simulink model "Xbox_collision_final"  (R2018b)
settings: Solver=FixedStepAuto  StartTime=0.0  StopTime=inf  FixedStep=Ts  RelTol=1e-3  EnableMultiTasking=on
PreLoadFcn:
  | config
InitFcn:
  | gb_params_obs
values from neighbouring files (symbols this model uses):
  A1 = [0, 0, 1, 0 ... (first row only)    [gb_load.m]    (also in gb_params_obs.m; model.m)
  A2 = [0   1 ... (first row only)    [gb_load.m]    (also in gb_params_obs.m; model.m)
  ag = 0.8    [gb_load.m]    (also in gb_params_obs.m; model.m)
  B1 = [0;0;2*alpha*(g2+g4)/g5; -2*alpha*(g2+g3)/g5]    [gb_load.m]    (also in gb_params_obs.m; model.m)
  B2 = [0 ... (first row only)    [gb_load.m]    (also in gb_params_obs.m; model.m)
  C1 = eye(4)    [gb_load.m]    (also in gb_params_obs.m; model.m = [1, -1, 0, 0)
  C1o = [1, -1, 0, 0 ... (first row only)    [gb_load.m]    (also in gb_params_obs.m)
  C2 = eye(2)    [gb_load.m]    (also in gb_params_obs.m; model.m = [1,0])
  C2o = [1,0]    [gb_load.m]    (also in gb_params_obs.m)
  Cg = [0,0,0,1,0,0]    [gb_load.m]    (also in gb_params_obs.m; model.m)
  Cm = [1,-1,0,0,1,0 ... (first row only)    [gb_load.m]    (also in gb_params_obs.m; model.m = [1,-1,0,0,W/(2*R),0)
  D1 = zeros(4, 1)    [gb_load.m]    (also in gb_params_obs.m)
  D2 = zeros(2,1)    [gb_load.m]    (also in gb_params_obs.m)
  EV3 = 0    [setup.m]
  K1i = lqrd(A1i, B1i, Q1i, R1i, Ts)    [gb_load.m]    (also in gb_params_obs.m)
  K2 = A2(2,2)^2/(4*B2(2,1))    [gb_load.m]    (also in gb_params_obs.m)
  kest = ss(ssd.A - L2t*ssd.C, [ssd.B L2t], ssd.C, zeros(2,3))    [gb_params_obs.m]
  R = 0.027    [gb_load.m]    (also in gb_params_obs.m; model.m; paramsCW2_v8.m = 0.01)
  Ts = 0.002    [gb_load.m]    (also in gb_params_obs.m; model.m; paramsCW2_v8.m = 0.004)
undefined symbols (not defined in the file or in its folder): DiscIntNeverNeededParam
libraries: legoev3lib x7, simulink_extras x6, simulink x1, shared_linuxserviceslib x1
settings Model: SimulationMode=external  ExtModeTrigDuration=2  Creator=thh206  LastModifiedBy=gazea
settings SolverCC: PositivePriorityOrder=on
settings OptimizationCC: EnhancedBackFolding=on  PassReuseOutputArgsAs=Individual arguments  MaxStackSize=64  OptimizeBlockOrder=speed  DifferentSizesBufferReuse=on  OptimizationCustomize=off
settings DebuggingCC: ParameterTunabilityLossMsg=error  LibraryContextMissingDiagnostic=none
settings HardwareCC: ProdBitPerPointer=32  ProdBitPerSizeT=32  ProdBitPerPtrDiffT=32  ProdLargestAtomicInteger=Long  ProdWordSize=32  ProdHWDeviceType=ARM Compatible->ARM 9
settings SFSimCC: SimUseLocalCustomCode=off  MATLABDynamicMemAlloc=off
settings RTWCC: SystemTargetFile=ert.tlc  HardwareBoard=LEGO MINDSTORMS EV3  TLCOptions="-aInlineSetEventsForThisBaseRateFcn=TLC_FALSE -aSuppressMultiTaskScheduler=TLC_FALSE  -aRateBasedStepFcn=0"  TemplateMakefile=ert_default_tmf  GenerateReport=on  RTWUseLocalCustomCode=off  Toolchain=Sourcery G++ Lite v2009q3  IncludeHyperlinkInReport=on  LaunchReport=on  GenerateTraceInfo=on  GenerateTraceReport=on  GenerateTraceReportSl=on  GenerateTraceReportSf=on  GenerateTraceReportEml=on
settings CodeAppCC: ForceParamTrailComments=on  IgnoreCustomStorageClasses=off  OperatorAnnotations=on  SimulinkDataObjDesc=on  SFDataObjDesc=on  InsertBlockDesc=on
settings ERTTargetCC: SupportContinuousTime=on  SupportVariableSizeSignals=on

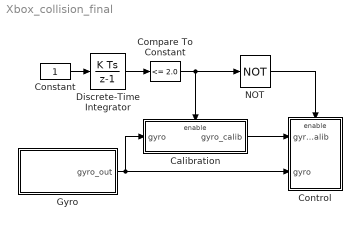
== system Xbox_collision_final ==
  Calibration : Subsystem
  Compare To Constant : simulink/Logic and Bit Operations/Compare To Constant  relop=<=  const=2.0  OutDataTypeStr=boolean
  Constant : Constant
  Control : Subsystem
  Discrete-Time Integrator : DiscreteIntegrator  SampleTime=Ts  ICPrevOutput=DiscIntNeverNeededParam  ICPrevScaledInput=DiscIntNeverNeededParam
  Gyro : Subsystem  Variant=on  VariantControl=Variant1
  NOT : Logic  Operator=NOT  IconShape=distinctive  AllPortsSameDT=off  OutDataTypeStr=boolean
  wires:
  Gyro/1(" gyro_out") -> Calibration/1(gyro), Control/2(gyro)
  Discrete-Time Integrator/1 -> Compare To Constant/1
  Compare To Constant/1 -> Calibration/Enable, NOT/1
  Constant/1 -> Discrete-Time Integrator/1
  NOT/1 -> Control/Enable
  Calibration/1(gyro_calib) -> Control/1(gyro_calib)

== system Xbox_collision_final/Calibration ==
  gyro : Inport
  Enable : EnablePort
  Gain1 : Gain  Gain=1-ag  OutDataTypeStr=Inherit: Same as input  ParamDataTypeStr=Inherit: Same as input
  Gain4 : Gain  Gain=ag  OutDataTypeStr=Inherit: Same as input  ParamDataTypeStr=Inherit: Same as input
  Scope : Scope
  Sum : Sum  Inputs=|++  OutDataTypeStr=Inherit: Same as first input
  Unit Delay : UnitDelay  InitialCondition=[0]  SampleTime=Ts
  gyro_calib : Outport
  wires:
  Unit Delay/1 -> Gain4/1
  Gain4/1 -> Sum/1
  Gain1/1 -> Sum/2
  Sum/1 -> Scope/1, gyro_calib/1, Unit Delay/1
  gyro/1 -> Gain1/1

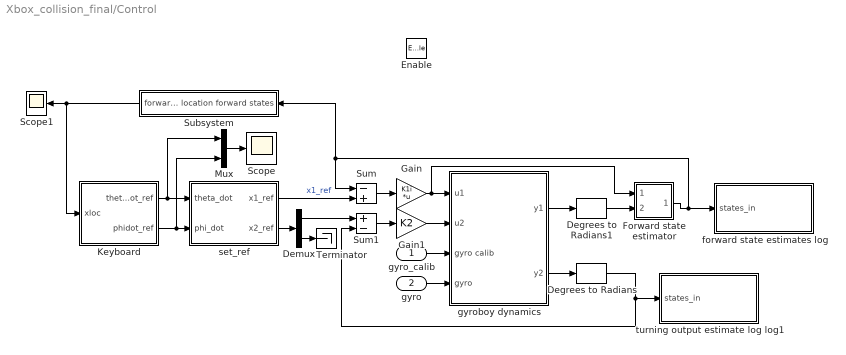
== system Xbox_collision_final/Control ==
  gyro_calib : Inport
  gyro : Inport  Port=2
  Enable : EnablePort
  Degrees to Radians : simulink_extras/Transformations/Degrees to Radians
  Degrees to Radians1 : simulink_extras/Transformations/Degrees to Radians
  Demux : Demux  Outputs=2
  Forward state estimator : Subsystem
  Gain : Gain  Gain=K1i  Multiplication=Matrix(K*u)
  Gain1 : Gain  Gain=K2
  Keyboard : Subsystem
  Mux : Mux  Inputs=2
  Scope : Scope
  Scope1 : Scope
  Subsystem : Subsystem
  Sum : Sum  Inputs=-+
  Sum1 : Sum  Inputs=+-
  Terminator : Terminator
  forward state estimates log : Subsystem  Variant=on  VariantControl=Variant1
  gyroboy dynamics : Subsystem  Variant=on  VariantControl=Variant1
  set_ref : Subsystem
  turning output estimate log log1 : Subsystem  Variant=on  VariantControl=Variant1
  wires:
  Keyboard/2(phidot_ref) -> Mux/2, set_ref/2(phi_dot)
  Keyboard/1(thetadot_ref) -> Mux/1, set_ref/1(theta_dot)
  Degrees to Radians/1 -> turning output estimate log log1/1(states_in), Sum1/2
  Gain/1 -> Forward state estimator/1(u1), gyroboy dynamics/1(u1)
  Gain1/1 -> gyroboy dynamics/2(u2)
  Sum1/1 -> Gain1/1
  gyroboy dynamics/2(y2) -> Degrees to Radians/1
  Mux/1 -> Scope/1
  set_ref/2(x2_ref) -> Demux/1
  Degrees to Radians1/1 -> Forward state estimator/2(y1)
  gyroboy dynamics/1(y1) -> Degrees to Radians1/1
  Demux/1 -> Sum1/1
  Sum/1 -> Gain/1
  Forward state estimator/1(x1e) -> forward state estimates log/1(states_in), Subsystem/1(forward states), Sum/1
  Demux/2 -> Terminator/1
  set_ref/1(x1_ref) -> Sum/2  "x1_ref"
  gyro_calib/1 -> gyroboy dynamics/3(gyro calib)
  Subsystem/1(forward location) -> Keyboard/1(xloc), Scope1/1
  gyro/1 -> gyroboy dynamics/4(gyro)

== system Xbox_collision_final/Gyro ==
  EV3 : Subsystem  VariantControl=HW == 1
  State-space : Subsystem  VariantControl=(default)
  " gyro_out" : Outport

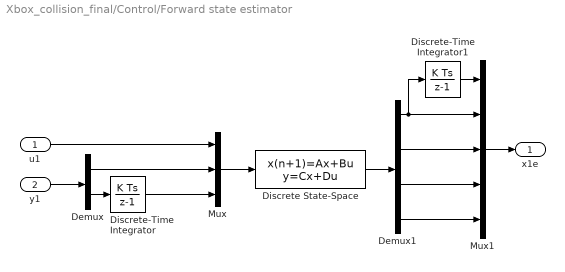
== system Xbox_collision_final/Control/Forward state estimator ==
  u1 : Inport
  y1 : Inport  Port=2
  Demux : Demux  Outputs=2
  Demux1 : Demux
  Discrete State-Space : DiscreteStateSpace  A=kest.A  B=kest.B  C=eye(4)  D=zeros(4,3)  InitialCondition=[0;0;0;0]  SampleTime=Ts
  Discrete-Time Integrator : DiscreteIntegrator  SampleTime=Ts  ICPrevOutput=DiscIntNeverNeededParam  ICPrevScaledInput=DiscIntNeverNeededParam
  Discrete-Time Integrator1 : DiscreteIntegrator  SampleTime=Ts  ICPrevOutput=DiscIntNeverNeededParam  ICPrevScaledInput=DiscIntNeverNeededParam
  Mux : Mux  Inputs=3
  Mux1 : Mux  Inputs=5
  x1e : Outport
  wires:
  y1/1 -> Demux/1
  Demux/2 -> Discrete-Time Integrator/1
  Discrete-Time Integrator/1 -> Mux/3
  Demux/1 -> Mux/2
  u1/1 -> Mux/1
  Mux/1 -> Discrete State-Space/1
  Demux1/4 -> Mux1/5
  Discrete-Time Integrator1/1 -> Mux1/1
  Demux1/1 -> Mux1/2, Discrete-Time Integrator1/1
  Demux1/2 -> Mux1/3
  Demux1/3 -> Mux1/4
  Mux1/1 -> x1e/1
  Discrete State-Space/1 -> Demux1/1

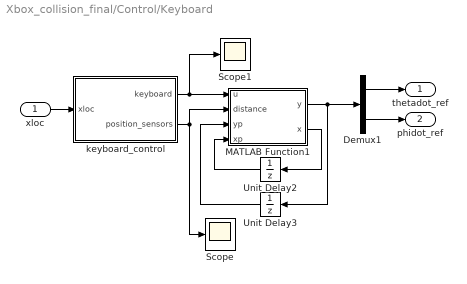
== system Xbox_collision_final/Control/Keyboard ==
  xloc : Inport
  Demux1 : Demux  Outputs=2
  MATLAB Function1 : MATLAB Function  TreatAsAtomicUnit=on
  Scope : Scope
  Scope1 : Scope
  Unit Delay2 : UnitDelay  InitialCondition=[0;0]  SampleTime=-1
  Unit Delay3 : UnitDelay  InitialCondition=[0;0]  SampleTime=-1
  keyboard_control : Subsystem  Variant=on  VariantControl=Variant1
  thetadot_ref : Outport
  phidot_ref : Outport  Port=2
  wires:
  Demux1/1 -> thetadot_ref/1
  MATLAB Function1/1(y) -> Demux1/1, Unit Delay3/1
  Unit Delay3/1 -> MATLAB Function1/3(yp)
  MATLAB Function1/2(x) -> Unit Delay2/1
  Unit Delay2/1 -> MATLAB Function1/4(xp)
  Demux1/2 -> phidot_ref/1
  keyboard_control/2(position_sensors) -> MATLAB Function1/2(distance), Scope/1
  keyboard_control/1(keyboard) -> MATLAB Function1/1(u), Scope1/1
  xloc/1 -> keyboard_control/1(xloc)

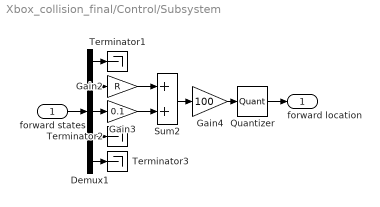
== system Xbox_collision_final/Control/Subsystem ==
  forward states : Inport
  Demux1 : Demux  Outputs=5
  Gain2 : Gain  Gain=R
  Gain3 : Gain  Gain=0.1
  Gain4 : Gain  Gain=100
  Quantizer : Quantizer  QuantizationInterval=1
  Sum2 : Sum
  Terminator1 : Terminator
  Terminator2 : Terminator
  Terminator3 : Terminator
  forward location : Outport
  wires:
  Demux1/3 -> Gain3/1
  Gain4/1 -> Quantizer/1
  Gain3/1 -> Sum2/2
  Sum2/1 -> Gain4/1
  Demux1/4 -> Terminator2/1
  Demux1/5 -> Terminator3/1
  Gain2/1 -> Sum2/1
  Demux1/1 -> Terminator1/1
  Demux1/2 -> Gain2/1
  Quantizer/1 -> forward location/1
  forward states/1 -> Demux1/1

== system Xbox_collision_final/Control/forward state estimates log ==
  states_in : Inport
  EV3 : Subsystem  VariantControl=HW == 1
  State-space : Subsystem  VariantControl=(default)

== system Xbox_collision_final/Control/gyroboy dynamics ==
  u1 : Inport
  u2 : Inport  Port=2
  gyro calib : Inport  Port=3
  gyro : Inport  Port=4
  EV3 : Subsystem  VariantControl=HW == 1
  State-space : Subsystem  VariantControl=(default)
  y1 : Outport
  y2 : Outport  Port=2

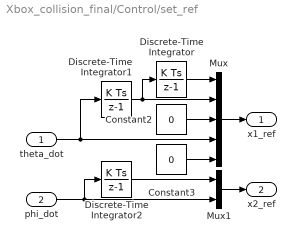
== system Xbox_collision_final/Control/set_ref ==
  theta_dot : Inport
  phi_dot : Inport  Port=2
  Constant2 : Constant  Value=0
  Constant3 : Constant  Value=0
  Discrete-Time Integrator : DiscreteIntegrator  SampleTime=-1  ICPrevOutput=DiscIntNeverNeededParam  ICPrevScaledInput=DiscIntNeverNeededParam
  Discrete-Time Integrator1 : DiscreteIntegrator  SampleTime=-1  ICPrevOutput=DiscIntNeverNeededParam  ICPrevScaledInput=DiscIntNeverNeededParam
  Discrete-Time Integrator2 : DiscreteIntegrator  SampleTime=-1  ICPrevOutput=DiscIntNeverNeededParam  ICPrevScaledInput=DiscIntNeverNeededParam
  Mux : Mux  Inputs=5
  Mux1 : Mux  Inputs=2
  x1_ref : Outport
  x2_ref : Outport  Port=2
  wires:
  Constant2/1 -> Mux/3
  Constant3/1 -> Mux/5
  Mux/1 -> x1_ref/1
  Discrete-Time Integrator1/1 -> Mux/2, Discrete-Time Integrator/1
  phi_dot/1 -> Mux1/2, Discrete-Time Integrator2/1
  Discrete-Time Integrator2/1 -> Mux1/1
  Discrete-Time Integrator/1 -> Mux/1
  theta_dot/1 -> Mux/4, Discrete-Time Integrator1/1
  Mux1/1 -> x2_ref/1

== system Xbox_collision_final/Control/turning output estimate log log1 ==
  states_in : Inport
  EV3 : Subsystem  VariantControl=HW == 1
  State-space : Subsystem  VariantControl=(default)

== system Xbox_collision_final/Gyro/EV3 ==
  Data Type Conversion1 : DataTypeConversion  OutDataTypeStr=double
  Gain : Gain  Gain=-1
  Gyro Sensor : legoev3lib/Gyro Sensor  portNumber=2  sampleTime=Ts
      settings: SourceProductName=Simulink Support Package for LEGO MINDSTORMS EV3 Hardware  SourceProductBaseCode=LEGOEV3
  gyro_out : Outport
  wires:
  Gyro Sensor/1 -> Data Type Conversion1/1
  Data Type Conversion1/1 -> Gain/1
  Gain/1 -> gyro_out/1

== system Xbox_collision_final/Gyro/State-space ==
  Constant : Constant  Value=4.0
  gyro_out : Outport
  wires:
  Constant/1 -> gyro_out/1

== system Xbox_collision_final/Control/Keyboard/keyboard_control ==
  xloc : Inport
  EV3 : Subsystem  VariantControl=HW == 1
  State-space : Subsystem  VariantControl=(default)
  keyboard : Outport
  position_sensors : Outport  Port=2

== system Xbox_collision_final/Control/forward state estimates log/EV3 ==
  states_in : Inport
  Forward states estimates : Scope
  wires:
  states_in/1 -> Forward states estimates/1

== system Xbox_collision_final/Control/forward state estimates log/State-space ==
  states_in : Inport
  Forward states estimates : Scope
  wires:
  states_in/1 -> Forward states estimates/1

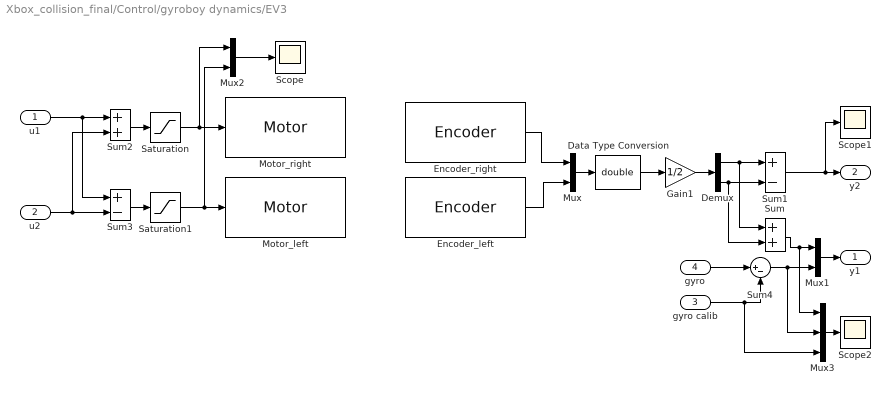
== system Xbox_collision_final/Control/gyroboy dynamics/EV3 ==
  u1 : Inport
  u2 : Inport  Port=2
  gyro calib : Inport  Port=3
  gyro : Inport  Port=4
  Data Type Conversion : DataTypeConversion  OutDataTypeStr=double
  Demux : Demux  Outputs=2
  Encoder_left : legoev3lib/Encoder  portNumber=D  opMode=No reset  sampleTime=Ts
      settings: SourceProductName=Simulink Support Package for LEGO MINDSTORMS EV3 Hardware  SourceProductBaseCode=LEGOEV3
  Encoder_right : legoev3lib/Encoder  portNumber=A  opMode=No reset  sampleTime=Ts
      settings: SourceProductName=Simulink Support Package for LEGO MINDSTORMS EV3 Hardware  SourceProductBaseCode=LEGOEV3
  Gain1 : Gain  Gain=1/2
  Motor_left : legoev3lib/Motor  sportNumber=D  sstopAction=Brake
  Motor_right : legoev3lib/Motor  sportNumber=A  sstopAction=Brake
  Mux : Mux  Inputs=2
  Mux1 : Mux  Inputs=2
  Mux2 : Mux  Inputs=2
  Mux3 : Mux  Inputs=3
  Saturation : Saturate  UpperLimit=100  LowerLimit=-100
  Saturation1 : Saturate  UpperLimit=100  LowerLimit=-100
  Scope : Scope
  Scope1 : Scope
  Scope2 : Scope
  Sum : Sum
  Sum1 : Sum  Inputs=+-
  Sum2 : Sum
  Sum3 : Sum  Inputs=+-
  Sum4 : Sum  Inputs=|+-
  y1 : Outport
  y2 : Outport  Port=2
  wires:
  u1/1 -> Sum3/1, Sum2/1
  Saturation/1 -> Mux2/1, Motor_right/1
  u2/1 -> Sum2/2, Sum3/2
  Saturation1/1 -> Mux2/2, Motor_left/1
  Mux/1 -> Data Type Conversion/1
  Encoder_right/1 -> Mux/1
  Encoder_left/1 -> Mux/2
  Data Type Conversion/1 -> Gain1/1
  Gain1/1 -> Demux/1
  Demux/1 -> Sum/1, Sum1/1
  Demux/2 -> Sum/2, Sum1/2
  Mux1/1 -> y1/1
  Sum/1 -> Mux3/1, Mux1/1
  gyro/1 -> Sum4/1
  gyro calib/1 -> Mux3/3, Sum4/2
  Sum4/1 -> Mux3/2, Mux1/2
  Mux2/1 -> Scope/1
  Sum1/1 -> Scope1/1, y2/1
  Mux3/1 -> Scope2/1
  Sum3/1 -> Saturation1/1
  Sum2/1 -> Saturation/1

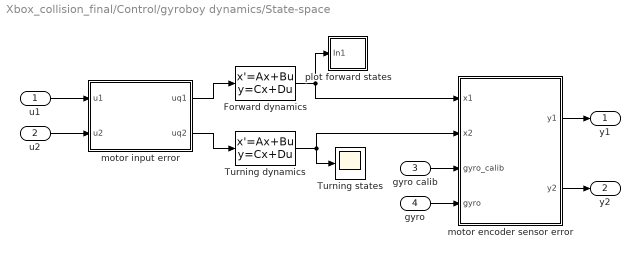
== system Xbox_collision_final/Control/gyroboy dynamics/State-space ==
  u1 : Inport
  u2 : Inport  Port=2
  gyro calib : Inport  Port=3
  gyro : Inport  Port=4
  Forward dynamics : StateSpace  A=A1  B=B1  C=C1  D=D1  InitialCondition=[0;0;0;0]
  Turning dynamics : StateSpace  A=A2  B=B2  C=C2  D=D2  InitialCondition=[0;0]
  Turning states : Scope
  motor encoder sensor error : Subsystem  Variant=on  VariantControl=Variant1
  motor input error : Subsystem  Variant=on  VariantControl=Variant1
  plot forward states : Subsystem
  y1 : Outport
  y2 : Outport  Port=2
  wires:
  u1/1 -> motor input error/1("u1 ")
  u2/1 -> motor input error/2(u2)
  motor encoder sensor error/1(" y1") -> y1/1
  motor input error/2(uq2) -> Turning dynamics/1
  motor encoder sensor error/2(" y2") -> y2/1
  motor input error/1(" uq1") -> Forward dynamics/1
  Forward dynamics/1 -> motor encoder sensor error/1("x1 "), plot forward states/1(In1)
  Turning dynamics/1 -> motor encoder sensor error/2(x2), Turning states/1
  gyro calib/1 -> motor encoder sensor error/3(gyro_calib)
  gyro/1 -> motor encoder sensor error/4(gyro)

== system Xbox_collision_final/Control/turning output estimate log log1/EV3 ==
  states_in : Inport
  Scope1 : Scope
  wires:
  states_in/1 -> Scope1/1

== system Xbox_collision_final/Control/turning output estimate log log1/State-space ==
  states_in : Inport
  Forward states estimates : Scope
  wires:
  states_in/1 -> Forward states estimates/1

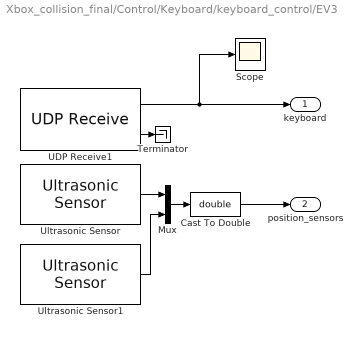
== system Xbox_collision_final/Control/Keyboard/keyboard_control/EV3 ==
  Cast To Double : DataTypeConversion  OutDataTypeStr=double
  Mux : Mux  Inputs=2
  Scope : Scope
  Terminator : Terminator
  UDP Receive1 : shared_linuxserviceslib/UDP Receive  localURL='0.0.0.0'  localPort=25000  remoteURL='0.0.0.0'  remotePort=-1  recvBufferSize=8192  signalDatatype=double  dims=2  isVarSize=off  showBlockingTime=off  blockingTime=0  sampletime=Ts  blockPlatform=LEGO EV3
  Ultrasonic Sensor : legoev3lib/Ultrasonic Sensor  PortNumber=1  sampleTime=Ts
      settings: SourceProductName=Simulink Support Package for LEGO MINDSTORMS EV3 Hardware  SourceProductBaseCode=LEGOEV3
  Ultrasonic Sensor1 : legoev3lib/Ultrasonic Sensor  PortNumber=3  sampleTime=Ts
      settings: SourceProductName=Simulink Support Package for LEGO MINDSTORMS EV3 Hardware  SourceProductBaseCode=LEGOEV3
  keyboard : Outport
  position_sensors : Outport  Port=2
  wires:
  Ultrasonic Sensor/1 -> Mux/1
  Ultrasonic Sensor1/1 -> Mux/2
  Mux/1 -> Cast To Double/1
  UDP Receive1/2 -> Terminator/1
  Cast To Double/1 -> position_sensors/1
  UDP Receive1/1 -> Scope/1, keyboard/1

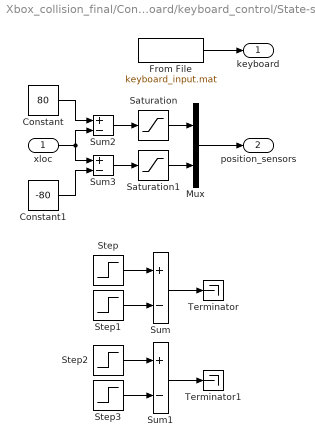
== system Xbox_collision_final/Control/Keyboard/keyboard_control/State-space ==
  xloc : Inport
  Constant : Constant  Value=80
  Constant1 : Constant  Value=-80
  From File : FromFile  FileName=keyboard_input.mat  SampleTime=0
  Mux : Mux  Inputs=2
  Saturation : Saturate  UpperLimit=255  LowerLimit=0
  Saturation1 : Saturate  UpperLimit=255  LowerLimit=0
  Step : Step  After=6  SampleTime=0
  Step1 : Step  Time=5  After=6  SampleTime=0
  Step2 : Step  Time=10  After=0.4  SampleTime=0
  Step3 : Step  Time=12  After=0.4  SampleTime=0
  Sum{,1..3} (4 alike) : Sum  Inputs=+-
  Terminator : Terminator
  Terminator1 : Terminator
  keyboard : Outport
  position_sensors : Outport  Port=2
  wires:
  Step1/1 -> Sum/2
  Sum/1 -> Terminator/1
  Step/1 -> Sum/1
  Step3/1 -> Sum1/2
  Sum1/1 -> Terminator1/1
  Step2/1 -> Sum1/1
  From File/1 -> keyboard/1
  Mux/1 -> position_sensors/1
  Constant/1 -> Sum2/1
  xloc/1 -> Sum3/1, Sum2/2
  Constant1/1 -> Sum3/2
  Sum2/1 -> Saturation/1
  Saturation1/1 -> Mux/2
  Sum3/1 -> Saturation1/1
  Saturation/1 -> Mux/1

== system Xbox_collision_final/Control/gyroboy dynamics/State-space/motor encoder sensor error ==
  "x1 " : Inport
  x2 : Inport  Port=2
  gyro_calib : Inport  Port=3
  gyro : Inport  Port=4
  ideal sensors : Subsystem  VariantControl=(default)
  sensor quantisation and saturation : Subsystem  VariantControl=real_model == 1
  " y1" : Outport
  " y2" : Outport  Port=2

== system Xbox_collision_final/Control/gyroboy dynamics/State-space/motor input error ==
  "u1 " : Inport
  u2 : Inport  Port=2
  ideal motor : Subsystem  VariantControl=(default)
  motor quantisation and saturation : Subsystem  VariantControl=real_model == 1
  " uq1" : Outport
  uq2 : Outport  Port=2

== system Xbox_collision_final/Control/gyroboy dynamics/State-space/plot forward states ==
  In1 : Inport
  Demux1 : Demux
  Discrete-Time Integrator : DiscreteIntegrator  SampleTime=Ts  ICPrevOutput=DiscIntNeverNeededParam  ICPrevScaledInput=DiscIntNeverNeededParam
  Forward states : Scope
  Mux2 : Mux  Inputs=5
  wires:
  Demux1/4 -> Mux2/5
  Demux1/3 -> Mux2/4
  In1/1 -> Demux1/1
  Mux2/1 -> Forward states/1
  Demux1/1 -> Mux2/2, Discrete-Time Integrator/1
  Demux1/2 -> Mux2/3
  Discrete-Time Integrator/1 -> Mux2/1

== system Xbox_collision_final/Control/gyroboy dynamics/State-space/motor encoder sensor error/ideal sensors ==
  "x1 " : Inport
  x2 : Inport  Port=2
  Gain : Gain  Gain=C1o  Multiplication=Matrix(K*u)
  Gain1 : Gain  Gain=C2o  Multiplication=Matrix(K*u)
  Radians to Degrees : simulink_extras/Transformations/Radians to Degrees
  Radians to Degrees1 : simulink_extras/Transformations/Radians to Degrees
  " y1" : Outport
  y2 : Outport  Port=2
  wires:
  "x1 "/1 -> Radians to Degrees/1
  Gain/1 -> " y1"/1
  x2/1 -> Radians to Degrees1/1
  Gain1/1 -> y2/1
  Radians to Degrees/1 -> Gain/1
  Radians to Degrees1/1 -> Gain1/1

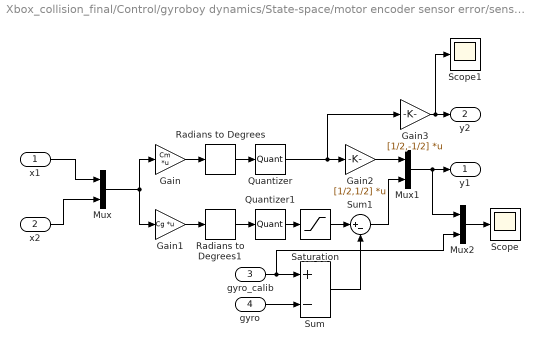
== system Xbox_collision_final/Control/gyroboy dynamics/State-space/motor encoder sensor error/sensor quantisation and saturation ==
  "x1 " : Inport
  x2 : Inport  Port=2
  gyro_calib : Inport  Port=3
  gyro : Inport  Port=4
  Gain : Gain  Gain=Cm  Multiplication=Matrix(K*u)
  Gain1 : Gain  Gain=Cg  Multiplication=Matrix(K*u)
  Gain2 : Gain  Gain=[1/2,1/2]  Multiplication=Matrix(K*u)
  Gain3 : Gain  Gain=[1/2,-1/2]  Multiplication=Matrix(K*u)
  Mux : Mux  Inputs=2
  Mux1 : Mux  Inputs=2
  Mux2 : Mux  Inputs=2
  Quantizer : Quantizer  QuantizationInterval=1
  Quantizer1 : Quantizer  QuantizationInterval=1
  Radians to Degrees : simulink_extras/Transformations/Radians to Degrees
  Radians to Degrees1 : simulink_extras/Transformations/Radians to Degrees
  Saturation : Saturate  UpperLimit=500  LowerLimit=-500
  Scope : Scope
  Scope1 : Scope
  Sum : Sum  Inputs=+-
  Sum1 : Sum  Inputs=|+-
  " y1" : Outport
  y2 : Outport  Port=2
  wires:
  Quantizer1/1 -> Saturation/1
  "x1 "/1 -> Mux/1
  x2/1 -> Mux/2
  Radians to Degrees/1 -> Quantizer/1
  Mux/1 -> Gain1/1, Gain/1
  Gain1/1 -> Radians to Degrees1/1
  Quantizer/1 -> Gain3/1, Gain2/1
  Gain2/1 -> Mux1/1
  Gain3/1 -> Scope1/1, y2/1
  Mux1/1 -> Mux2/1, " y1"/1
  Gain/1 -> Radians to Degrees/1
  Radians to Degrees1/1 -> Quantizer1/1
  gyro_calib/1 -> Mux2/2, Sum/1
  gyro/1 -> Sum/2
  Saturation/1 -> Sum1/1
  Sum1/1 -> Mux1/2
  Sum/1 -> Sum1/2
  Mux2/1 -> Scope/1

== system Xbox_collision_final/Control/gyroboy dynamics/State-space/motor input error/ideal motor ==
  "u1 " : Inport
  u2 : Inport  Port=2
  " uq1" : Outport
  uq2 : Outport  Port=2
  wires:
  "u1 "/1 -> " uq1"/1
  u2/1 -> uq2/1

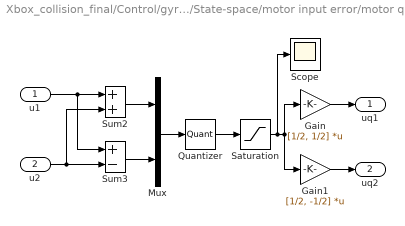
== system Xbox_collision_final/Control/gyroboy dynamics/State-space/motor input error/motor quantisation and saturation ==
  "u1 " : Inport
  u2 : Inport  Port=2
  Gain : Gain  Gain=[1/2, 1/2]  Multiplication=Matrix(K*u)
  Gain1 : Gain  Gain=[1/2, -1/2]  Multiplication=Matrix(K*u)
  Mux : Mux  Inputs=2
  Quantizer : Quantizer  QuantizationInterval=1
  Saturation : Saturate  UpperLimit=100  LowerLimit=-100
  Scope : Scope
  Sum2 : Sum
  Sum3 : Sum  Inputs=+-
  " uq1" : Outport
  uq2 : Outport  Port=2
  wires:
  Saturation/1 -> Scope/1, Gain1/1, Gain/1
  Sum2/1 -> Mux/1
  u2/1 -> Sum2/2, Sum3/2
  Quantizer/1 -> Saturation/1
  Sum3/1 -> Mux/2
  Mux/1 -> Quantizer/1
  "u1 "/1 -> Sum3/1, Sum2/1
  Gain/1 -> " uq1"/1
  Gain1/1 -> uq2/1

== matlab function Xbox_collision_final/Control/Keyboard/MATLAB Function1 ==
  data: u input; distance input; y output; yp input; xp input; x output
function [y,x] = fcn(u, distance, yp, xp)
maxController = 127; % maximum controller input
u = u/maxController; % normalise inputs
x = xp;
y = yp;
thetadotref = yp(1);
phidotref = yp(2);
acctheta = abs(4*0.002*u(1)); %increment in theta in one time step (0.002s)
thetadotmax = abs(8*u(1));
phidotmax = abs(1.2*u(2)); %increment in phi in one time step (0.002s)

% Retreat from object in front of gyroboy
if x(1) == 2
    if distance(1) < 50
        u(1) = -1;
    else
        x(1) = 4;
    end
end

% Retreat from object behind gyroboy
if x(1) == 3
    if distance(2) < 50
        u(1) = 1;
    else
        x(1) = 5;
    end
end

% Overrides keyboard input - makes gyroboy stop after retreating from
% object
if x(1) == 4
    if u(1) == 1
        u(1) = 0;
    else
        x(1) = 1;
    end
end

if x(1) == 5
    if u(1) == -1
        u(1) = 0;
    else
        x(1) = 1;
    end
end

% Collision detection
if distance(1) < 25
   x(1) = 2;
   u(1) = -1;
end

if distance(2) < 25
   x(1) = 3;
   u(1) = 1;
end 

% if up was pressed, accelerate
if u(1) > 0
    if thetadotref < thetadotmax
        thetadotref = thetadotref + acctheta;
    else
        thetadotref = thetadotmax;
    end
end

% if down was pressed, decelerate
if u(1) < 0
    if thetadotref > -thetadotmax
        thetadotref = thetadotref - acctheta;
    else
        thetadotref = -thetadotmax;
    end
end

% space = stop
if u(1) == 0
    if thetadotref > (0 + acctheta/2)
        thetadotref = thetadotref - acctheta;
    elseif thetadotref < (0 - acctheta/2)
        thetadotref = thetadotref + acctheta;
    else
        thetadotref = 0;
    end;
end

% turning left
if u(2) > 0
    phidotref = -phidotmax;
end

% turning right
if u(2) < 0
    phidotref = phidotmax;
end

% stop
if u(2) == 0
    phidotref = 0;
end

y = [thetadotref; phidotref];
end
